simulink model "Final_Simulink_Model"  (R2022b)
settings: Solver=FixedStepAuto  StartTime=0.0  StopTime=10.0  FixedStep=1e-3  RelTol=1e-3  EnableMultiTasking=on
undefined symbols (not defined in the file): D0, D1, D10, D11, D12, D13, D2, D3, D4, D5, D6, D7, D8, D9, PTA0, PTA1, PTA2, PTB23, PTB9, PTC16, PTC17, PTC2, PTC3, PTC4, PTD0, PTD1, PTD2, PTD3
libraries: frdmk64flib x14
settings Model: ExtModeTrigDuration=5  Creator=clara  LastModifiedBy=clara
settings OptimizationCC: EnhancedBackFolding=on  PassReuseOutputArgsAs=Individual arguments  ZeroExternalMemoryAtStartup=off  ZeroInternalMemoryAtStartup=off  MaxStackSize=64  OptimizeBlockOrder=speed  DifferentSizesBufferReuse=on  OptimizationCustomize=off  EfficientTunableParamExpr=on
settings DebuggingCC: ParameterTunabilityLossMsg=error
settings HardwareCC: ProdBitPerPointer=32  ProdBitPerSizeT=32  ProdBitPerPtrDiffT=32  ProdLargestAtomicInteger=Long  ProdLargestAtomicFloat=Double  ProdWordSize=32  ProdHWDeviceType=ARM Compatible->ARM Cortex
settings ModelReferenceCC: EnableRefExpFcnMdlSchedulingChecks=on
settings SFSimCC: MATLABDynamicMemAlloc=off
settings RTWCC: Description=Embedded Coder  SystemTargetFile=ert.tlc  HardwareBoard=NXP FRDM-K64F  TLCOptions="-aInlineSetEventsForThisBaseRateFcn=TLC_FALSE -aSuppressMultiTaskScheduler=TLC_FALSE  -aRateBasedStepFcn=0"  TemplateMakefile=ert_default_tmf  Toolchain=GNU Tools for ARM Embedded Processors
settings CodeAppCC: ForceParamTrailComments=on  IgnoreCustomStorageClasses=off  OperatorAnnotations=on  SimulinkDataObjDesc=on  SFDataObjDesc=on  InsertBlockDesc=on
settings ERTTargetCC: ExtModeTransport=4  ExtModeMexFile=sendToCommService

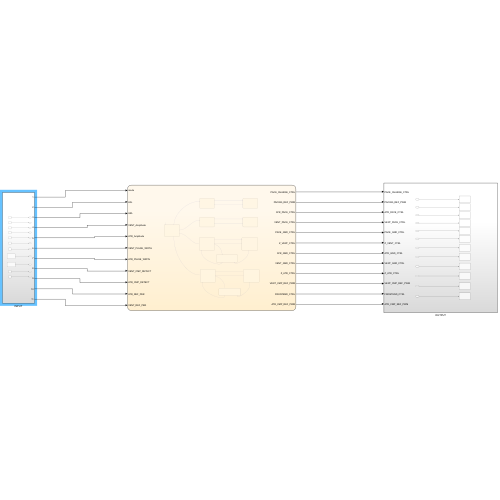
[thumbnail: Simulink's stored preview of the top-level diagram]
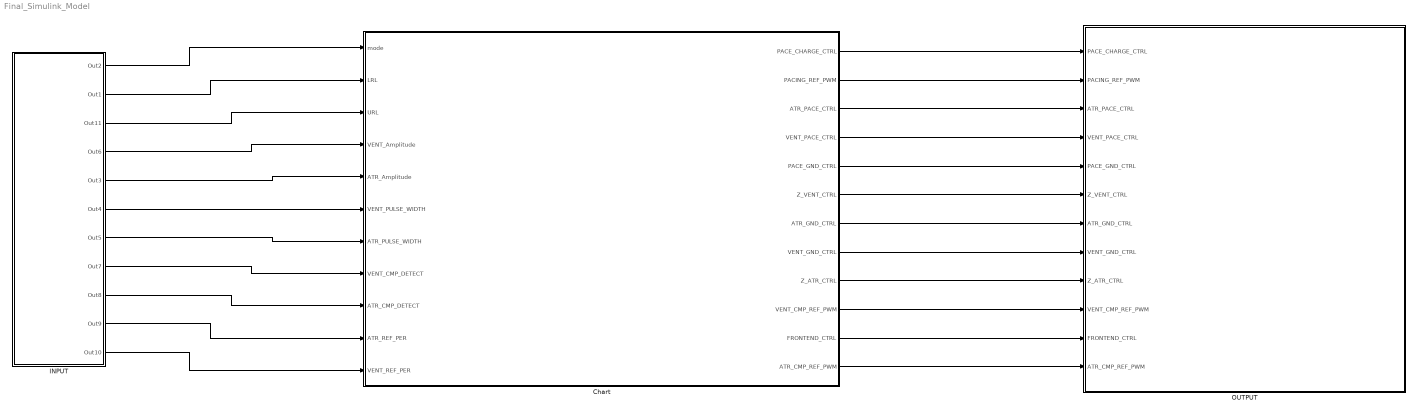
== system Final_Simulink_Model ==
  Chart : Stateflow chart  TreatAsAtomicUnit=on
      settings: PortSchema="{\"entries\":[{\"content\":{\"sides\":[{\"content\":{\"connectorIds\":[\"In10\",\"In1\",\"In6\",\"In2\",\"In3\",\"In4\",\"In5\",\"In7\",\"In8\",\"In9\",\"In11\"]},\"type\":\"ConnectorPlacement.EquallySpacedRectSide\",\"uuid\":\"411cfc43-89c3-4653-9fab-0da98be593d3\"},{\"content\":{\"connectorIds\":[\"Out1\",\"Out2\",\"Out3\",\"Out4\",\"Out5\",\"Out6\",\"Out7\",\"Out8\",\"Out9\",\"Out10\",\"Out11\",\"Out12\"],\"side\":\"RIGHT\"},\"type\":\"ConnectorPlacement.EquallySpacedRectSide\",\"uuid\":\"ad1683f7-26aa-4767-b656-f3b731cb8235\"},{\"content\":{\"connectorIds\":[],\"side\":\"TOP\"},\"type\":\"ConnectorPlacement.EquallySpacedRectSide\",\"uuid\":\"fbccba07-c1cc-4c9f-8e56-0bdfb6912bb8\"}]},\"type\":\"ConnectorPlacement.EquallySpacedConnector\",\"uuid\":\"0c618a7f-9484-4de3-a6ac-3c8308721375\"}],\"packageUris\":[\"http://schema.mathworks.com/mf0/Connector/R2020b\"],\"version\":\"1.0\"}"
  "INPUT " : Subsystem
  OUTPUT : Subsystem
  wires:
  Chart/7(ATR_GND_CTRL) -> OUTPUT/7(ATR_GND_CTRL)
  Chart/3(ATR_PACE_CTRL) -> OUTPUT/3(ATR_PACE_CTRL)
  Chart/6(Z_VENT_CTRL) -> OUTPUT/6(Z_VENT_CTRL)
  Chart/8(VENT_GND_CTRL) -> OUTPUT/8(VENT_GND_CTRL)
  Chart/5(PACE_GND_CTRL) -> OUTPUT/5(PACE_GND_CTRL)
  Chart/9(Z_ATR_CTRL) -> OUTPUT/9(Z_ATR_CTRL)
  Chart/2(PACING_REF_PWM) -> OUTPUT/2(PACING_REF_PWM)
  Chart/1(PACE_CHARGE_CTRL) -> OUTPUT/1(PACE_CHARGE_CTRL)
  Chart/4(VENT_PACE_CTRL) -> OUTPUT/4(VENT_PACE_CTRL)
  Chart/11(FRONTEND_CTRL) -> OUTPUT/11(FRONTEND_CTRL)
  Chart/10(VENT_CMP_REF_PWM) -> OUTPUT/10(VENT_CMP_REF_PWM)
  "INPUT "/1(Out2) -> Chart/10(mode)
  "INPUT "/2(Out1) -> Chart/1(LRL)
  "INPUT "/3(Out11) -> Chart/6(URL)
  "INPUT "/4(Out6) -> Chart/2(VENT_Amplitude)
  "INPUT "/5(Out3) -> Chart/3(ATR_Amplitude)
  "INPUT "/6(Out4) -> Chart/4(VENT_PULSE_WIDTH)
  "INPUT "/7(Out5) -> Chart/5(ATR_PULSE_WIDTH)
  "INPUT "/8(Out7) -> Chart/7(VENT_CMP_DETECT)
  "INPUT "/9(Out8) -> Chart/8(ATR_CMP_DETECT)
  Chart/12(ATR_CMP_REF_PWM) -> OUTPUT/12(ATR_CMP_REF_PWM)
  "INPUT "/10(Out9) -> Chart/9(ATR_REF_PER)
  "INPUT "/11(Out10) -> Chart/11(VENT_REF_PER)

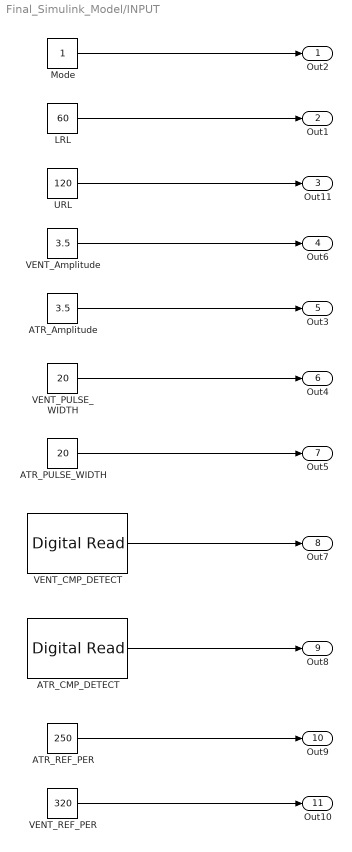
== system Final_Simulink_Model/INPUT  ==
  ATR_Amplitude : Constant  Value=3.5
  ATR_CMP_DETECT : frdmk64flib/Digital Read  Whichpin=PTC16 (D0)  SampleTime=-1
  ATR_PULSE_WIDTH : Constant  Value=20
  ATR_REF_PER : Constant  Value=250
  LRL : Constant  Value=60
  Mode : Constant
  URL : Constant  Value=120
  VENT_Amplitude : Constant  Value=3.5
  VENT_CMP_DETECT : frdmk64flib/Digital Read  Whichpin=PTC17 (D1)  SampleTime=-1
  VENT_PULSE_WIDTH : Constant  Value=20
  VENT_REF_PER : Constant  Value=320
  Out2 : Outport
  Out1 : Outport  Port=2
  Out11 : Outport  Port=3
  Out6 : Outport  Port=4
  Out3 : Outport  Port=5
  Out4 : Outport  Port=6
  Out5 : Outport  Port=7
  Out7 : Outport  Port=8
  Out8 : Outport  Port=9
  Out9 : Outport  Port=10
  Out10 : Outport  Port=11
  wires:
  LRL/1 -> Out1/1
  VENT_PULSE_WIDTH/1 -> Out4/1
  VENT_Amplitude/1 -> Out6/1
  URL/1 -> Out11/1
  Mode/1 -> Out2/1
  ATR_Amplitude/1 -> Out3/1
  ATR_PULSE_WIDTH/1 -> Out5/1
  VENT_CMP_DETECT/1 -> Out7/1
  ATR_CMP_DETECT/1 -> Out8/1
  ATR_REF_PER/1 -> Out9/1
  VENT_REF_PER/1 -> Out10/1

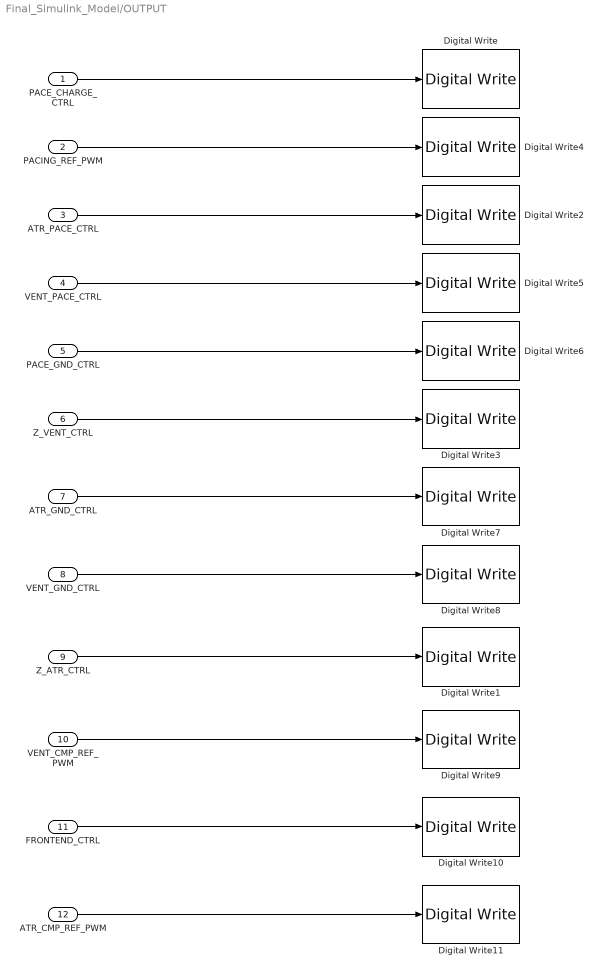
== system Final_Simulink_Model/OUTPUT ==
  PACE_CHARGE_CTRL : Inport
  PACING_REF_PWM : Inport  Port=2
  ATR_PACE_CTRL : Inport  Port=3
  VENT_PACE_CTRL : Inport  Port=4
  PACE_GND_CTRL : Inport  Port=5
  Z_VENT_CTRL : Inport  Port=6
  ATR_GND_CTRL : Inport  Port=7
  VENT_GND_CTRL : Inport  Port=8
  Z_ATR_CTRL : Inport  Port=9
  VENT_CMP_REF_PWM : Inport  Port=10
  FRONTEND_CTRL : Inport  Port=11
  ATR_CMP_REF_PWM : Inport  Port=12
  Digital Write : frdmk64flib/Digital Write  Whichpin=PTB9 (D2)
  Digital Write1 : frdmk64flib/Digital Write  Whichpin=PTB23 (D4)
  Digital Write10 : frdmk64flib/Digital Write  Whichpin=PTD1 (D13)
  Digital Write11 : frdmk64flib/Digital Write  Whichpin=PTC2 (D6)
  Digital Write2 : frdmk64flib/Digital Write  Whichpin=PTA0 (D8)
  Digital Write3 : frdmk64flib/Digital Write  Whichpin=PTC3 (D7)
  Digital Write4 : frdmk64flib/Digital Write  Whichpin=PTA2 (D5)
  Digital Write5 : frdmk64flib/Digital Write  Whichpin=PTC4 (D9)
  Digital Write6 : frdmk64flib/Digital Write  Whichpin=PTD0 (D10)
  Digital Write7 : frdmk64flib/Digital Write  Whichpin=PTD2 (D11)
  Digital Write8 : frdmk64flib/Digital Write  Whichpin=PTD3 (D12)
  Digital Write9 : frdmk64flib/Digital Write  Whichpin=PTA1 (D3)
  wires:
  PACE_CHARGE_CTRL/1 -> Digital Write/1
  PACING_REF_PWM/1 -> Digital Write4/1
  ATR_PACE_CTRL/1 -> Digital Write2/1
  VENT_PACE_CTRL/1 -> Digital Write5/1
  PACE_GND_CTRL/1 -> Digital Write6/1
  Z_VENT_CTRL/1 -> Digital Write3/1
  ATR_GND_CTRL/1 -> Digital Write7/1
  VENT_GND_CTRL/1 -> Digital Write8/1
  Z_ATR_CTRL/1 -> Digital Write1/1
  VENT_CMP_REF_PWM/1 -> Digital Write9/1
  FRONTEND_CTRL/1 -> Digital Write10/1
  ATR_CMP_REF_PWM/1 -> Digital Write11/1

== stateflow chart Final_Simulink_Model/Chart ==
  note: Pace ready
  state AOO
    entry:
    % charge condition for C22
    ATR_PACE_CTRL = false;
    VENT_PACE_CTRL = false;
    PACE_CHARGE_CTRL = true;
    % discharge condition for C21;
    ATR_GND_CTRL = true;
    PACE_GND_CTRL = true;
    VENT_GND_CTRL = false;
    Z_ATR_CTRL = false;
    Z_VENT_CTRL = false;
    %
    PACING_REF_PWM = 20*ATR_Amplitude;
  state Pacing_AOO
    entry:
    PACE_CHARGE_CTRL = false;
    PACE_GND_CTRL = true;
    ATR_PACE_CTRL = true;
    ATR_GND_CTRL = false;
    Z_ATR_CTRL = false;
    Z_VENT_CTRL = false;
    VENT_GND_CTRL = false;
    VENT_PACE_CTRL = false;
    %
  note: Recharge ready
  note: Charge C22 and discharge blocking capacitor
  note: Discharge C22 into atrium (charge C21)
  note: Pace ready
  state VOO
    entry:
    % charge condition for C22
    ATR_PACE_CTRL = false;
    VENT_PACE_CTRL = false;
    PACE_CHARGE_CTRL = true;
    % discharge condition for C21;
    VENT_GND_CTRL = true;
    PACE_GND_CTRL = true;
    ATR_GND_CTRL = false;
    Z_ATR_CTRL = false;
    Z_VENT_CTRL = false;
    %
    PACING_REF_PWM = 20*VENT_Amplitude;
  state Pacing_VOO
    entry:
    PACE_CHARGE_CTRL = false;
    PACE_GND_CTRL = true;
    ATR_PACE_CTRL = false;
    ATR_GND_CTRL = false;
    Z_ATR_CTRL = false;
    Z_VENT_CTRL = false;
    VENT_GND_CTRL = false;
    VENT_PACE_CTRL = true;
    %
  note: Initial conditions
  state MAIN
    entry:
    VENT_GND_CTRL=false;
    Z_ATR_CTRL = false;
    Z_VENT_CTRL = false;
    FRONTEND_CTRL=false;
    PACE_CHARGE_CTRL = false;
    VENT_PACE_CTRL = false;
    ATR_PACE_CTRL = false;
    PACE_GND_CTRL=false;
    ATR_GND_CTRL=false;
  note: Recharge ready
  note: Charge C22 and discharge blocking capacitor
  note: Discharge C22 into ventrical (charge C21)
  note: Begin sensing, charge C22 and discharge
      | blocking capacitor
  note: Discharge C22 into atrium (charge C21)
  note: If no signal is sensed
  state AAI
    entry:
    % begin sensing
    FRONTEND_CTRL = true;
    % charge condition for C22
    ATR_PACE_CTRL = false;
    VENT_PACE_CTRL = false;
    PACE_CHARGE_CTRL = true;
    % discharge condition for C21;
    ATR_GND_CTRL = true;
    PACE_GND_CTRL = true;
    VENT_GND_CTRL = false;
    Z_ATR_CTRL = false;
    Z_VENT_CTRL = false;
    %
    PACING_REF_PWM = 20*ATR_Amplitude;
    ATR_CMP_REF_PWM = 20*ATR_Amplitude;
  state Pacing_VVI1
    entry:
    PACE_CHARGE_CTRL = false;
    PACE_GND_CTRL = true;
    ATR_PACE_CTRL = true;
    ATR_GND_CTRL = false;
    Z_ATR_CTRL = false;
    Z_VENT_CTRL = false;
    VENT_GND_CTRL = false;
    VENT_PACE_CTRL = false;
    %
    PACING_REF_PWM = 20*ATR_Amplitude;
  note: If signal is sensed
  state AAI_REFRACTORY
    entry:
    FRONTEND_CTRL = false;
    ATR_PACE_CTRL = false;
    VENT_PACE_CTRL = false;
    ATR_GND_CTRL = true;
    PACING_REF_PWM = 20*ATR_Amplitude;
    PACE_CHARGE_CTRL = false;
    PACE_GND_CTRL = true;
  note: If signal is sensed
  note: Follows events during which senses
      | in the atrium are ignored
  note: Begin sensing, charge C22 and discharge
      | blocking capacitor
  note: Discharge C22 into ventrical (charge C21)
  note: If no signal is sensed
  state VVI
    entry:
    % begin sensing
    FRONTEND_CTRL = true;
    % charge condition for C22
    ATR_PACE_CTRL = false;
    VENT_PACE_CTRL = false;
    PACE_CHARGE_CTRL = true;
    % discharge condition for C21;
    VENT_GND_CTRL = true;
    PACE_GND_CTRL = true;
    ATR_GND_CTRL = false;
    Z_ATR_CTRL = false;
    Z_VENT_CTRL = false;
    %
    PACING_REF_PWM = 20*VENT_Amplitude;
    VENT_CMP_REF_PWM = 20*VENT_Amplitude;
  state Pacing_VVI
    entry:
    PACE_CHARGE_CTRL = false;
    PACE_GND_CTRL = true;
    ATR_PACE_CTRL = false;
    ATR_GND_CTRL = false;
    Z_ATR_CTRL = false;
    Z_VENT_CTRL = false;
    VENT_GND_CTRL = false;
    VENT_PACE_CTRL = true;
    %
    PACING_REF_PWM = 20*VENT_Amplitude;
  note: If signal is sensed
  state VVI_REFRACTORY
    entry:
    FRONTEND_CTRL = false;
    ATR_PACE_CTRL = false;
    VENT_GND_CTRL = true;
    PACING_REF_PWM = 20*VENT_Amplitude;
    PACE_CHARGE_CTRL = false;
    PACE_GND_CTRL = true;
  note: If signal is sensed
  note: Follows events during which senses
      | in the ventrical are ignored
  AOO -> Pacing_AOO : [after(60000/LRL - ATR_PULSE_WIDTH,msec)]
  MAIN -> AOO [order 4] : [mode == 1]
  Pacing_AOO -> AOO : [after(ATR_PULSE_WIDTH,msec)]
  VOO -> Pacing_VOO : [after(60000/LRL - VENT_PULSE_WIDTH,msec)]
  MAIN -> VOO [order 1] : [mode == 2]
  (default) -> MAIN
  Pacing_VOO -> VOO : [after(VENT_PULSE_WIDTH,msec)]
  MAIN -> AAI [order 3] : [mode == 3]
  MAIN -> VVI [order 2] : [mode == 4]
  AAI -> Pacing_VVI1 [order 1] : [(ATR_CMP_DETECT==false) &&after(60000/LRL - ATR_PULSE_WIDTH,msec)]
  Pacing_VVI1 -> AAI [order 1] : [after(ATR_PULSE_WIDTH,msec)]
  AAI -> AAI_REFRACTORY [order 2] : [ATR_CMP_DETECT == true]
  AAI_REFRACTORY -> AAI
  Pacing_VVI1 -> AAI_REFRACTORY [order 2] : [ATR_CMP_DETECT == true]
  VVI -> Pacing_VVI [order 1] : [(VENT_CMP_DETECT==false) &&after(60000/LRL - VENT_PULSE_WIDTH,msec)]
  Pacing_VVI -> VVI [order 1] : [after(VENT_PULSE_WIDTH,msec)]
  VVI -> VVI_REFRACTORY [order 2] : [VENT_CMP_DETECT == true]
  VVI_REFRACTORY -> VVI
  Pacing_VVI -> VVI_REFRACTORY [order 2] : [VENT_CMP_DETECT == true]
  data: LRL input; VENT_Amplitude input; ATR_Amplitude input; VENT_PULSE_WIDTH input; ATR_PULSE_WIDTH input; URL input; VENT_CMP_DETECT input; ATR_CMP_DETECT input; ATR_REF_PER input; PACE_CHARGE_CTRL output; PACING_REF_PWM output; ATR_PACE_CTRL output; VENT_PACE_CTRL output; PACE_GND_CTRL output; Z_VENT_CTRL output; ATR_GND_CTRL output; VENT_GND_CTRL output; Z_ATR_CTRL output; VENT_CMP_REF_PWM output; FRONTEND_CTRL output; mode input; ATR_CMP_REF_PWM output; VENT_REF_PER input
